simulink model "BilinearTransformation"  (R2020b)
settings: Solver=VariableStepAuto  StartTime=0.0  StopTime=10  RelTol=1e-3
settings Model: Creator=Shubham  LastModifiedBy=Shubham
settings DataIOCC: ExternalInput=[t, freq]  LoadExternalInput=on  SaveFormat=Array  ReturnWorkspaceOutputs=off  OutputSaveName=output

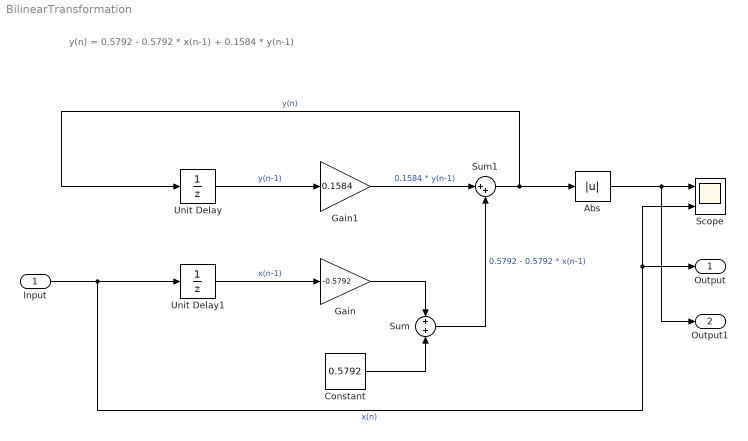
== system BilinearTransformation ==
  note: y(n) = 0.5792 - 0.5792 * x(n-1) + 0.1584 * y(n-1)
  Input : Inport
  Abs : Abs
  Constant : Constant  Value=0.5792
  Gain : Gain  Gain=-0.5792
  Gain1 : Gain  Gain=0.1584
  Scope : Scope  NumInputPorts=2
  Sum : Sum
  Sum1 : Sum  Inputs=|++
  Unit Delay : UnitDelay  SampleTime=-1  HasFrameUpgradeWarning=on
  Unit Delay1 : UnitDelay  SampleTime=-1  HasFrameUpgradeWarning=on
  Output : Outport
  Output1 : Outport  Port=2
  wires:
  Input/1 -> Unit Delay1/1, Scope/2, Output/1  "x(n)"
  Unit Delay1/1 -> Gain/1  "x(n-1)"
  Unit Delay/1 -> Gain1/1  "y(n-1)"
  Sum1/1 -> Abs/1, Unit Delay/1  "y(n)"
  Constant/1 -> Sum/2
  Gain/1 -> Sum/1
  Sum/1 -> Sum1/2  "0.5792 - 0.5792 * x(n-1)"
  Gain1/1 -> Sum1/1  "0.1584 * y(n-1)"
  Abs/1 -> Output1/1, Scope/1
